simulink model "TurtleModel"  (R2018b)
settings: Solver=FixedStepAuto  StartTime=0.0  StopTime=50  FixedStep=0.01  RelTol=1e-3
libraries: simulink x4
settings Model: Creator=DwigHT  LastModifiedBy=DwigHT

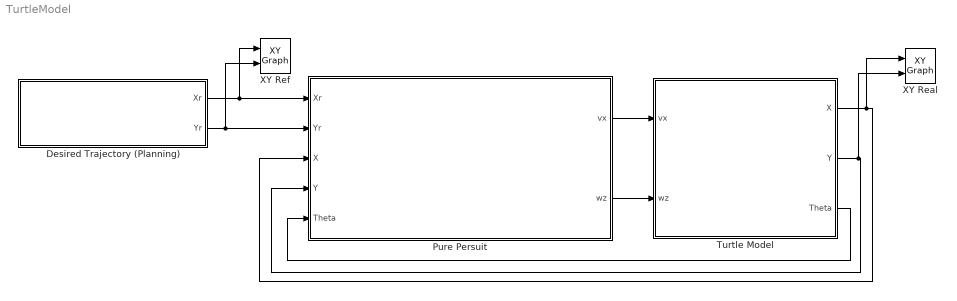
== system TurtleModel ==
  Desired Trajectory (Planning) : Subsystem
  Pure Persuit : Subsystem
  Turtle Model : Subsystem
  XY Real : simulink/Sinks/XY Graph  xmin=0  xmax=11  ymin=0  ymax=11  st=-1
  XY Ref : simulink/Sinks/XY Graph  xmin=0  xmax=11  ymin=0  ymax=11  st=-1
  wires:
  Desired Trajectory (Planning)/1(Xr) -> XY Ref/1, Pure Persuit/1(Xr)
  Desired Trajectory (Planning)/2(Yr) -> XY Ref/2, Pure Persuit/2(Yr)
  Turtle Model/2(Y) -> XY Real/2, Pure Persuit/4(Y)
  Turtle Model/1(X) -> XY Real/1, Pure Persuit/3(X)
  Turtle Model/3(Theta) -> Pure Persuit/5(Theta)
  Pure Persuit/1(vx) -> Turtle Model/1(vx)
  Pure Persuit/2(wz) -> Turtle Model/2(wz)

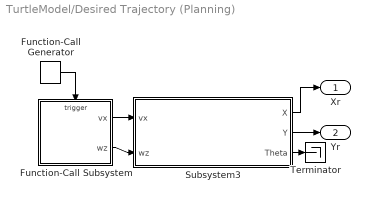
== system TurtleModel/Desired Trajectory (Planning) ==
  Function-Call Generator : simulink/Ports & Subsystems/Function-Call Generator  sample_time=1  numberOfIterations=1
  Function-Call Subsystem : Subsystem  TreatAsAtomicUnit=on
  Subsystem3 : Subsystem
  Terminator : Terminator
  Xr : Outport
  Yr : Outport  Port=2
  wires:
  Subsystem3/2(Y) -> Yr/1
  Subsystem3/3(Theta) -> Terminator/1
  Function-Call Subsystem/2(wz) -> Subsystem3/2(wz)
  Function-Call Subsystem/1(vx) -> Subsystem3/1(vx)
  Subsystem3/1(X) -> Xr/1
  Function-Call Generator/1 -> Function-Call Subsystem/Trigger

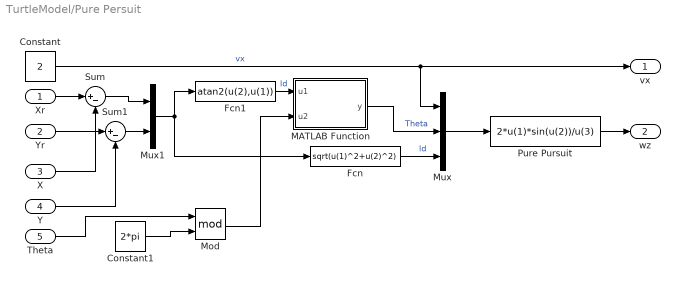
== system TurtleModel/Pure Persuit ==
  Xr : Inport
  Yr : Inport  Port=2
  X : Inport  Port=3
  Y : Inport  Port=4
  Theta : Inport  Port=5
  Constant : Constant  Value=2
  Constant1 : Constant  Value=2*pi
  Fcn : Fcn  Expr=sqrt(u(1)^2+u(2)^2)
  Fcn1 : Fcn  Expr=atan2(u(2),u(1))
  MATLAB Function : MATLAB Function  TreatAsAtomicUnit=on
  Mod : Math  Operator=mod  SaturateOnIntegerOverflow=on
  Mux : Mux  Inputs=3
  Mux1 : Mux  Inputs=2
  Pure Pursuit : Fcn  Expr=2*u(1)*sin(u(2))/u(3)
  Sum : Sum  Inputs=|+-
  Sum1 : Sum  Inputs=|+-
  vx : Outport
  wz : Outport  Port=2
  wires:
  Mux/1 -> Pure Pursuit/1
  Sum1/1 -> Mux1/2
  Fcn1/1 -> MATLAB Function/1(u1)  "ld"
  Constant/1 -> vx/1, Mux/1  "vx"
  X/1 -> Sum/2
  Mod/1 -> MATLAB Function/2(u2)
  Sum/1 -> Mux1/1
  MATLAB Function/1(y) -> Mux/2  "Theta"
  Mux1/1 -> Fcn1/1, Fcn/1
  Constant1/1 -> Mod/2
  Fcn/1 -> Mux/3  "ld"
  Pure Pursuit/1 -> wz/1
  Yr/1 -> Sum1/1
  Theta/1 -> Mod/1
  Xr/1 -> Sum/1
  Y/1 -> Sum1/2

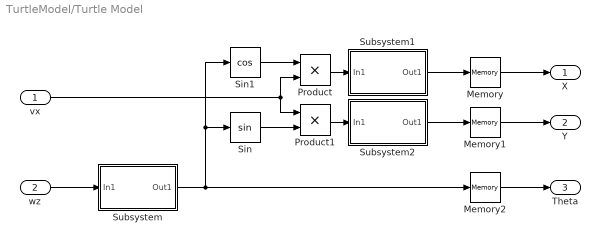
== system TurtleModel/Turtle Model ==
  vx : Inport
  wz : Inport  Port=2
  Memory : Memory  InitialCondition=5.55
  Memory1 : Memory  InitialCondition=5.55
  Memory2 : Memory
  Product : Product
  Product1 : Product
  Sin : Trigonometry
  Sin1 : Trigonometry  Operator=cos
  Subsystem : Subsystem
  Subsystem1 : Subsystem
  Subsystem2 : Subsystem
  X : Outport
  Y : Outport  Port=2
  Theta : Outport  Port=3
  wires:
  Product1/1 -> Subsystem2/1(In1)
  Subsystem2/1(Out1) -> Memory1/1
  Sin1/1 -> Product/1
  Subsystem1/1(Out1) -> Memory/1
  vx/1 -> Product/2, Product1/1
  Product/1 -> Subsystem1/1(In1)
  Subsystem/1(Out1) -> Memory2/1, Sin/1, Sin1/1
  Sin/1 -> Product1/2
  wz/1 -> Subsystem/1(In1)
  Memory/1 -> X/1
  Memory1/1 -> Y/1
  Memory2/1 -> Theta/1

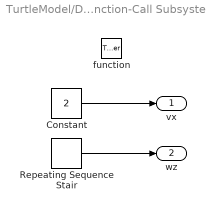
== system TurtleModel/Desired Trajectory (Planning)/Function-Call Subsystem ==
  function : TriggerPort  TriggerType=function-call  VariantControl=Variant
  Constant : Constant  Value=2
  Repeating Sequence Stair : simulink/Sources/Repeating Sequence Stair  OutValues=[1 2 3 2].'  tsamp=-1  OutMin=[]  OutMax=[]  OutDataTypeStr=double  OutputDataTypeScalingMode=double  OutDataType=fixdt(0,8)  ConRadixGroup=Best Precision: Vector-wise  OutScaling=2^-12
  vx : Outport
  wz : Outport  Port=2
  wires:
  Constant/1 -> vx/1
  Repeating Sequence Stair/1 -> wz/1

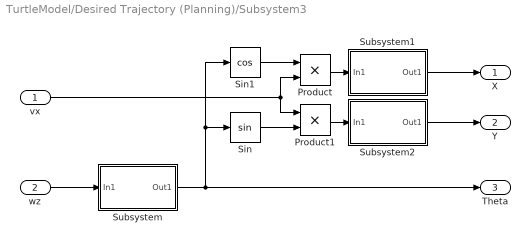
== system TurtleModel/Desired Trajectory (Planning)/Subsystem3 ==
  vx : Inport
  wz : Inport  Port=2
  Product : Product
  Product1 : Product
  Sin : Trigonometry
  Sin1 : Trigonometry  Operator=cos
  Subsystem : Subsystem
  Subsystem1 : Subsystem
  Subsystem2 : Subsystem
  X : Outport
  Y : Outport  Port=2
  Theta : Outport  Port=3
  wires:
  Product1/1 -> Subsystem2/1(In1)
  Subsystem2/1(Out1) -> Y/1
  Sin1/1 -> Product/1
  Subsystem1/1(Out1) -> X/1
  vx/1 -> Product/2, Product1/1
  Product/1 -> Subsystem1/1(In1)
  Subsystem/1(Out1) -> Theta/1, Sin/1, Sin1/1
  Sin/1 -> Product1/2
  wz/1 -> Subsystem/1(In1)

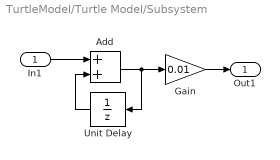
== system TurtleModel/Turtle Model/Subsystem ==
  In1 : Inport
  Add : Sum
  Gain : Gain  Gain=0.01
  Unit Delay : UnitDelay  SampleTime=0.01
  Out1 : Outport
  wires:
  Unit Delay/1 -> Add/2
  Add/1 -> Gain/1, Unit Delay/1
  Gain/1 -> Out1/1
  In1/1 -> Add/1

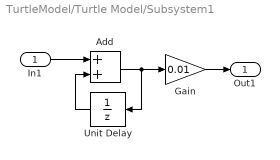
== system TurtleModel/Turtle Model/Subsystem1 ==
  In1 : Inport
  Add : Sum
  Gain : Gain  Gain=0.01
  Unit Delay : UnitDelay  InitialCondition=555  SampleTime=0.01
  Out1 : Outport
  wires:
  In1/1 -> Add/1
  Gain/1 -> Out1/1
  Add/1 -> Unit Delay/1, Gain/1
  Unit Delay/1 -> Add/2

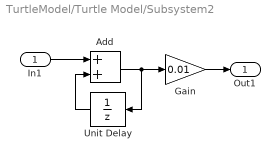
== system TurtleModel/Turtle Model/Subsystem2 ==
  In1 : Inport
  Add : Sum
  Gain : Gain  Gain=0.01
  Unit Delay : UnitDelay  InitialCondition=555  SampleTime=0.01
  Out1 : Outport
  wires:
  Unit Delay/1 -> Add/2
  Add/1 -> Gain/1, Unit Delay/1
  Gain/1 -> Out1/1
  In1/1 -> Add/1

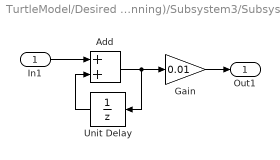
== system TurtleModel/Desired Trajectory (Planning)/Subsystem3/Subsystem ==
  In1 : Inport
  Add : Sum
  Gain : Gain  Gain=0.01
  Unit Delay : UnitDelay  SampleTime=0.01
  Out1 : Outport
  wires:
  Unit Delay/1 -> Add/2
  Add/1 -> Gain/1, Unit Delay/1
  Gain/1 -> Out1/1
  In1/1 -> Add/1

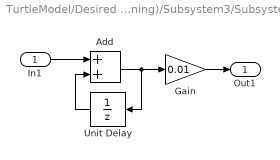
== system TurtleModel/Desired Trajectory (Planning)/Subsystem3/Subsystem1 ==
  In1 : Inport
  Add : Sum
  Gain : Gain  Gain=0.01
  Unit Delay : UnitDelay  InitialCondition=555  SampleTime=0.01
  Out1 : Outport
  wires:
  In1/1 -> Add/1
  Gain/1 -> Out1/1
  Add/1 -> Unit Delay/1, Gain/1
  Unit Delay/1 -> Add/2

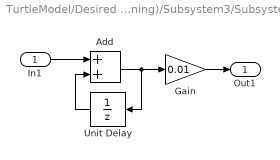
== system TurtleModel/Desired Trajectory (Planning)/Subsystem3/Subsystem2 ==
  In1 : Inport
  Add : Sum
  Gain : Gain  Gain=0.01
  Unit Delay : UnitDelay  InitialCondition=555  SampleTime=0.01
  Out1 : Outport
  wires:
  Unit Delay/1 -> Add/2
  Add/1 -> Gain/1, Unit Delay/1
  Gain/1 -> Out1/1
  In1/1 -> Add/1

== matlab function TurtleModel/Pure Persuit/MATLAB Function ==
  data: u1 input; y output; u2 input
function y = fcn(u1,u2)
if u1<0
    u1=u1+2*pi;
end
y = u1-u2;
